simulink model "Ex1"  (R2018a)
settings: Solver=VariableStepAuto  StartTime=0.0  StopTime=10  RelTol=1e-3
values from neighbouring files (symbols this model uses):
  b = 0.2    [Main_1_1.m]    (also in ScriptEx1Simulink.m)
  k = 2    [Main_1_1.m]    (also in ScriptEx1Simulink.m)
  m = 15    [Main_1_1.m]    (also in ScriptEx1Simulink.m)
settings Model: Creator=MSI User  LastModifiedBy=MSI User

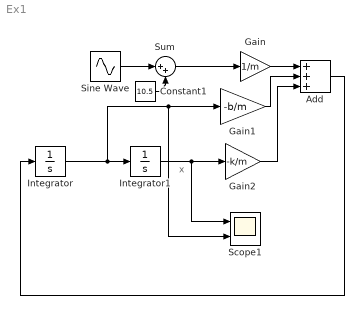
== system Ex1 ==
  note: x
  Add : Sum  Inputs=+++
  Constant1 : Constant  Value=10.5
  Gain : Gain  Gain=1/m
  Gain1 : Gain  Gain=-b/m
  Gain2 : Gain  Gain=-k/m
  Integrator : Integrator
  Integrator1 : Integrator
  Scope1 : Scope  NumInputPorts=2
  Sine Wave : Sin  Amplitude=5  Frequency=2  SampleTime=0
  Sum : Sum  Inputs=|++
  wires:
  Constant1/1 -> Sum/2
  Sum/1 -> Gain/1
  Gain/1 -> Add/1
  Gain1/1 -> Add/2
  Gain2/1 -> Add/3
  Integrator/1 -> Integrator1/1, Scope1/2, Gain1/1
  Integrator1/1 -> Scope1/1, Gain2/1
  Add/1 -> Integrator/1
  Sine Wave/1 -> Sum/1
